simulink model "temp_mmms4th"  (R2024b)
settings: Solver=VariableStepAuto  StartTime=0.0  StopTime=10.0  RelTol=1e-3
values from neighbouring files (symbols this model uses):
  iota0 = eye(6,6)    [Initiate_KUKA_inv.m]    (also in Main_MMMS.m; test_KUKA_elements.m)
  K_d = 10*[1.3*eye(3) zeros(3);zeros(3) 0.8*eye(3)]    [Initiate_FQ.m]    (also in Initiate_KUKA_inv.m = 5*[0.7*eye(3) zeros(3);zeros(3) 0.5*eye(3)]; MMMS_Initiate_FQ.m; Main_MMMS.m = 5*[0.7*eye(3) zeros(3);zeros(3) 0.5*eye(3)]; test_KUKA_elements.m = 50*[0.7*eye(3) zeros(3);zeros(3) 0.5*eye(3)])
  K_i = 5*[0.1*eye(3) zeros(3);zeros(3) 0.01*eye(3)]    [Initiate_FQ.m]    (also in Initiate_KUKA_inv.m = 5*[0.01*eye(3) zeros(3);zeros(3) 0.001*eye(3)]; MMMS_Initiate_FQ.m; Main_MMMS.m = 5*[0.01*eye(3) zeros(3);zeros(3) 0.001*eye(3)]; test_KUKA_elements.m = 50*[0.01*eye(3) zeros(3);zeros(3) 0.001*eye(3)])
  K_p = 100*[0.1 0 0 0 0 0;0 0.1 0 0 0 0; 0 0 0.1 0 0 0; 0 0 0 0.01 0 0 ... (first row only)    [Initiate_FQ.m]    (also in Initiate_KUKA_inv.m = 5*[0.1 0 0 0 0 0;0 0.1 0 0 0 0; 0 0 0.1 0 0 0; 0 0 0 0.01 0 ; MMMS_Initiate_FQ.m; Main_MMMS.m = 5*[0.1 0 0 0 0 0;0 0.1 0 0 0 0; 0 0 0.1 0 0 0; 0 0 0 0.01 0 ; test_KUKA_elements.m = 50*[0.1 0 0 0 0 0;0 0.1 0 0 0 0; 0 0 0.1 0 0 0; 0 0 0 0.01 0)
  K_w = 200*eye(7)    [Initiate_FQ.m]    (also in MMMS_Initiate_FQ.m)
  K_wd = 2*eye(7)    [Initiate_FQ.m]    (also in MMMS_Initiate_FQ.m)
  M0 = M_temp.M0.data(:,:,1)    [Initiate_FQ.m]    (also in MMMS_Initiate_FQ.m; test_KUKA_elements.m)
  m0_frak = diag_M(1:6,1:6)    [Initiate_KUKA_inv.m]    (also in Main_MMMS.m; make_uncertain.m = diag_M_unc(1:6,1:6); test_KUKA_elements.m)
  M0m = M_temp.M0m.data(:,:,1)    [Initiate_FQ.m]    (also in MMMS_Initiate_FQ.m; test_KUKA_elements.m)
  m_diag = diag_M(7:end,7:end)    [Initiate_KUKA_inv.m]    (also in Main_MMMS.m; make_uncertain.m = diag_M_unc(7:end,7:end); test_KUKA_elements.m)
  M_t = (((Adjoint(g_It))'\M_t_body)/(Adjoint(g_It)))    [Initiate_FQ.m]    (also in Initiate_KUKA_inv.m = [eye(3)*mt zeros(3); zeros(3) eye(3)*80]; MMMS_Initiate_FQ.m; Main_MMMS.m = [eye(3)*mt zeros(3); zeros(3) eye(3)*80]; test_KUKA_elements.m = [eye(3)*mt zeros(3); zeros(3) eye(3)*80])
  M_t_body = [eye(3)*mt zeros(3); zeros(3) eye(3)*0.416667]    [Initiate_FQ.m]    (also in MMMS_Initiate_FQ.m)
  mu = P0    [Initiate_FQ.m]    (also in Initiate_KUKA_inv.m = zeros(6,1); MMMS_Initiate_FQ.m; Main_MMMS.m = zeros(6,1); make_uncertain.m = P0_unc)
  mu_t = inv((Adjoint(g_It))')*M_t_body*[V_It;w_t]    [Initiate_FQ.m]    (also in Initiate_KUKA_inv.m = M_t*[V_0t;w_t]; MMMS_Initiate_FQ.m; Main_MMMS.m = M_t*[V_0t;w_t]; make_uncertain.m = inv((Adjoint(g_It))')*M_t_body_unc*[V_It;w_t])
  sc_size = 1    [Initiate_KUKA_inv.m]    (also in Main_MMMS.m; test_KUKA_elements.m)
  Xi_m_matrix = zeros(6*n,n)    [Initiate_KUKA_inv.m]    (also in Main_MMMS.m)
undefined symbols (not defined in the file or in its folder): Mm, Xi_m
(part 1 of 2)
settings Model: Creator=bmonazza  LastModifiedBy=bmonazza

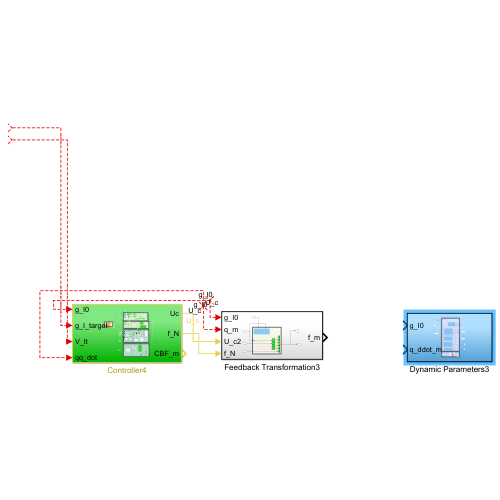
[thumbnail: Simulink's stored preview of the top-level diagram]
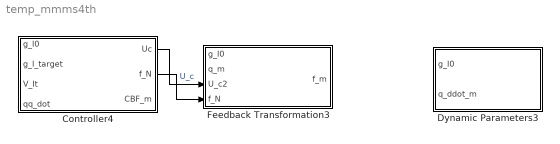
== system temp_mmms4th ==
  Controller4 : Subsystem
  Dynamic Parameters3 : Subsystem
  Feedback Transformation3 : Subsystem
  wires:
  ? -> Controller4/2(g_I_target)
  Controller4/1(Uc) -> Feedback Transformation3/3(U_c2)  "U_c"
  Controller4/2(f_N) -> Feedback Transformation3/4(f_N)
  ? -> Controller4/1(g_I0)  "g_I0"
  ? -> Feedback Transformation3/1(g_I0)  "g_I0"
  ? -> Feedback Transformation3/2(q_m)  "U_c"
  ? -> Controller4/3(V_It)
  ? -> Controller4/4(qq_dot)  "U_c"

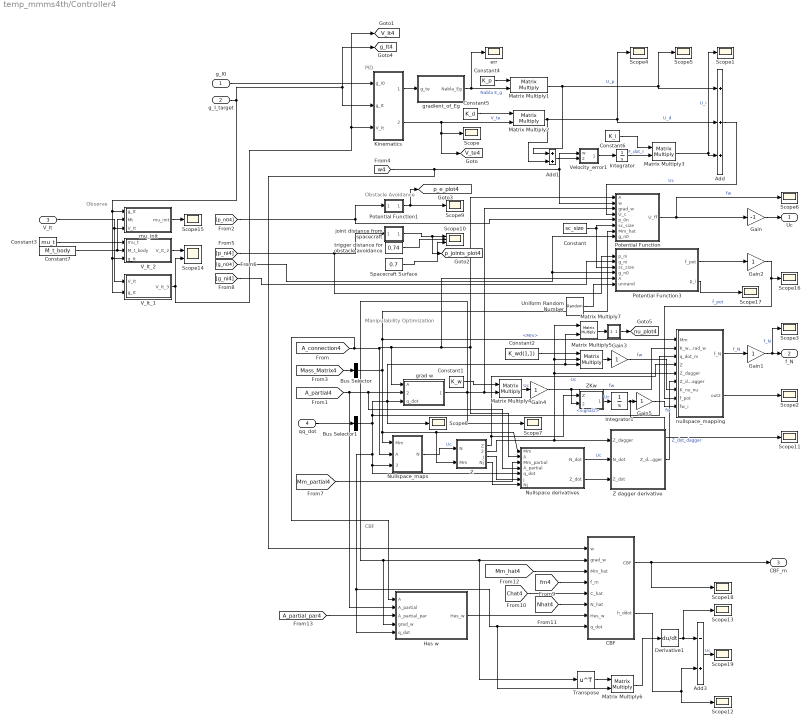
== system temp_mmms4th/Controller4 ==
  note: CBF
  note: Observe
  note: Obstacle Avoidance
  note: Manipulability Optimization
  note: PID
  g_I0 : Inport
  g_I_target : Inport  Port=2
  V_It : Inport  Port=3
  qq_dot : Inport  Port=4
  " " : MATLAB Function  TreatAsAtomicUnit=on
  Add : Sum  Inputs=+++
  Add1 : Sum
  Add3 : Sum  Inputs=-+
  Bus Selector : BusSelector  OutputSignals=Mm
  Bus Selector1 : BusSelector  OutputSignals=signal2
  CBF : MATLAB Function  TreatAsAtomicUnit=on
  Constant : Constant  Value=sc_size
  Constant1 : Constant  Value=K_w
  Constant2 : Constant  Value=K_wd(1,1)
  Constant3 : Constant  Value=mu_t
  Constant4 : Constant  Value=K_p
  Constant5 : Constant  Value=K_d
  Constant6 : Constant  Value=K_i
  Constant7 : Constant  Value=M_t_body
  Derivative1 : Derivative
  Gain : Gain  Gain=-1
  Gain{1..5} (5 alike) : Gain
  Hes w : MATLAB Function  TreatAsAtomicUnit=on
  Integrator : Integrator
  Integrator1 : Integrator
  Kinematics : Subsystem
  Matrix Multiply{1..4,6..7} (6 alike) : Product  Multiplication=Matrix(*)
  Matrix Multiply5 : Product  Inputs=3  Multiplication=Matrix(*)
  Nullspace derivatives : MATLAB Function  TreatAsAtomicUnit=on
  Nullspace_maps : MATLAB Function  TreatAsAtomicUnit=on
  Potential Function : MATLAB Function  TreatAsAtomicUnit=on
  Potential Function1 : MATLAB Function  TreatAsAtomicUnit=on
  Potential Function3 : MATLAB Function  TreatAsAtomicUnit=on
  Scope{,1..9,11..13,15..19} (18 alike) : Scope
  Scope10 : Scope  NumInputPorts=3
  Scope14 : Scope  NumInputPorts=2
  Spacecraft Surface : Constant  Value=0.7
  Transpose : Math  Operator=transpose
  Uniform Random Number : UniformRandomNumber  SampleTime=0.1
  V_It_1 : MATLAB Function  TreatAsAtomicUnit=on
  V_It_2 : MATLAB Function  TreatAsAtomicUnit=on
  Velocity_error1 : MATLAB Function  TreatAsAtomicUnit=on
  Z : MATLAB Function  TreatAsAtomicUnit=on
  Z dagger derivative : MATLAB Function  TreatAsAtomicUnit=on
  ZKw : MATLAB Function  TreatAsAtomicUnit=on
  err : Scope
  grad w : MATLAB Function  TreatAsAtomicUnit=on
  gradient_of_Eg : MATLAB Function  TreatAsAtomicUnit=on
  joint distance from spacecraft : MATLAB Function  TreatAsAtomicUnit=on
  mu_init : MATLAB Function  TreatAsAtomicUnit=on
  nullspace_mapping : MATLAB Function  TreatAsAtomicUnit=on
  trigger distance for obstacle avoidance : Constant  Value=0.74
  Uc : Outport
  f_N : Outport  Port=2
  CBF_m : Outport  Port=3
  tag scope: V_It4=global, V_te4=global, g_It4=global, nu_plot4=global, p_e_plot4=global, p_joints_plot4=global
  wires:
  Uniform Random Number/1 -> Potential Function3/6(unirand)
  [A_connection4] -> Hes w/1(A), Nullspace_maps/2(A), grad w/1(A), Nullspace derivatives/2(A), Potential Function/1(A), Potential Function3/5(A)
  [Chat4] -> CBF/5(C_hat)
  [Nhat4] -> CBF/6(N_hat)
  Derivative1/1 -> Add3/1, Scope13/1
  [A_partial_par4] -> Hes w/3(A_partial_par)
  Transpose/1 -> Matrix Multiply6/1
  Matrix Multiply6/1 -> Derivative1/1
  CBF/2(h_ddot) -> Scope12/1, Add3/2
  [Mm_hat4] -> CBF/3(Mm_hat)
  [fm4] -> CBF/4(f_m)
  Hes w/1(Hes_w) -> CBF/7(Hes_w)
  CBF/1(CBF) -> CBF_m/1, Scope18/1
  Add3/1 -> Scope19/1  "Uc"
  [w4] -> Velocity_error1/1(w), Potential Function/2(w), CBF/1(w)
  [A_partial4] -> Hes w/2(A_partial), Nullspace derivatives/4(A_partial), grad w/2(A_partial)
  Bus Selector1/1 -> Nullspace_maps/3(q_dot_m), Nullspace derivatives/5(q_dot), CBF/8(q_dot), Matrix Multiply6/2, Hes w/5(q_dot), Matrix Multiply5/3, Matrix Multiply7/2, grad w/3(q_dot), Scope8/1, nullspace_mapping/3(q_dot_m)  "<signal2>"
  grad w/1(grad_w) -> Matrix Multiply4/2, Potential Function/3(grad_w), Scope7/1, Hes w/4(grad_w), CBF/2(grad_w), Transpose/1
  Matrix Multiply7/1 -> " "/1(A)
  " "/1(normA) -> [nu_plot4]
  g_I_target/1 -> mu_init/1(g_It), V_It_2/3(g_It), V_It_1/2(g_It), [g_It4], Kinematics/2(g_It)
  Potential Function3/2(p_i) -> Scope17/1
  [g_ni4] -> Potential Function3/2(g_ni)
  Spacecraft Surface/1 -> Scope10/3
  V_It_1/1(V_It_3) -> [V_It4], Kinematics/3(V_It), Scope14/2
  V_It_2/1(V_It_2) -> Scope14/1
  Z/4(Nj) -> Nullspace derivatives/7(Nj)
  Z/3(j) -> Nullspace derivatives/6(j)
  Gain2/1 -> nullspace_mapping/8(f_pot), Scope16/1  "f_pot"
  Constant7/1 -> V_It_2/2(M_t_body), mu_init/2(Mt)
  mu_init/1(mu_init) -> Scope15/1
  Constant3/1 -> V_It_2/1(mu_t)
  V_It/1 -> mu_init/3(V_It), V_It_1/1(V_It)
  Gain5/1 -> nullspace_mapping/9(fw_i)  "fw"
  Integrator1/1 -> Gain5/1, Scope11/1
  ZKw/1(out) -> Integrator1/1  "Uc"
  Z/2(Z_dagger) -> Matrix Multiply5/2, Matrix Multiply7/1, nullspace_mapping/5(Z_dagger), Z dagger derivative/1(Z_dagger)
  nullspace_mapping/2(out2) -> Scope2/1
  Gain4/1 -> nullspace_mapping/2(K_w_grad_w), ZKw/2(K_w_grad_w)  "fw"
  Z/1(Z) -> nullspace_mapping/4(Z), ZKw/1(Z)  "Uc"
  [Mm_partial4] -> Nullspace derivatives/3(Mm_partial)
  Nullspace_maps/1(N) -> Z/1(N)  "Uc"
  Z dagger derivative/1(Z_dot_dagger) -> nullspace_mapping/6(Z_dot_dagger)  "Z_dot_dagger"
  Nullspace derivatives/2(Z_dot) -> Z dagger derivative/3(Z_dot)
  Nullspace derivatives/1(N_dot) -> Z dagger derivative/2(N_dot)  "Uc"
  Gain3/1 -> nullspace_mapping/7(K_nu_nu)  "fw"
  trigger distance for obstacle avoidance/1 -> Scope10/2
  Constant/1 -> Potential Function/6(sc_size), Potential Function3/3(sc_size)
  Potential Function3/1(f_pot) -> Gain2/1
  [g_n04] -> Potential Function/8(g_n0), Potential Function3/4(g_n0)
  joint distance from spacecraft/1(pnorm) -> Scope10/1, [p_joints_plot4]
  [p_ni4] -> Potential Function3/1(p_ni), joint distance from spacecraft/1(p_joints)
  Potential Function1/1(w_p) -> [p_e_plot4], Scope9/1
  [p_n04] -> Potential Function/5(p_0n), Potential Function1/1(p_0n)
  Velocity_error1/1(out) -> Integrator/1
  Potential Function/1(U_ff) -> Scope6/1, Gain/1  "fw"
  nullspace_mapping/1(f_N) -> Gain1/1  "f_N"
  Matrix Multiply3/1 -> Add/3, Scope1/1  "U_i"
  Matrix Multiply4/1 -> Gain4/1  "Uc"
  Constant2/1 -> Matrix Multiply5/1
  Matrix Multiply5/1 -> Gain3/1
  Constant1/1 -> Matrix Multiply4/1
  Gain1/1 -> Scope3/1, f_N/1  "f_N"
  Constant5/1 -> Matrix Multiply2/1
  Matrix Multiply1/1 -> Add1/1, Add/1, Scope5/1  "U_p"
  Integrator/1 -> Matrix Multiply3/2  "F_dot_I"
  Constant6/1 -> Matrix Multiply3/1
  Kinematics/2(V_te) -> Matrix Multiply2/2, Scope/1, [V_te4]  "V_te"
  Constant4/1 -> Matrix Multiply1/1
  gradient_of_Eg/1(Nabla_Eg) -> Matrix Multiply1/2, err/1  "Nabla E_g"
  Matrix Multiply2/1 -> Add1/2, Add/2, Scope4/1  "U_d"
  Add1/1 -> Velocity_error1/2(in)
  Kinematics/1(g_te1) -> gradient_of_Eg/1(g_te)
  Add/1 -> Potential Function/4(U_c)  "Uc"
  g_I0/1 -> Kinematics/1(g_I0)
  Gain/1 -> Uc/1
  Bus Selector/1 -> nullspace_mapping/1(Mm), Potential Function/7(Mm_hat), Nullspace derivatives/1(Mm), Z/2(Mm), Nullspace_maps/1(Mm)  "<Mm>"
  [Mass_Matrix4] -> Bus Selector/1
  qq_dot/1 -> Bus Selector1/1

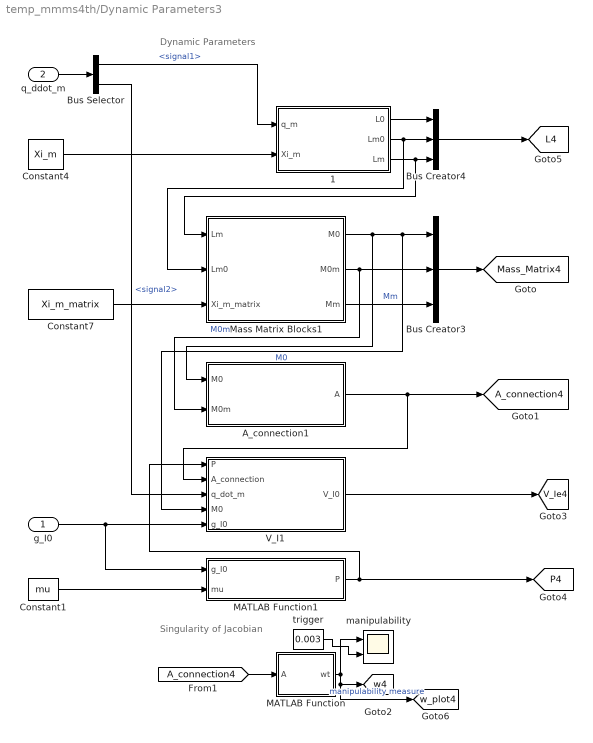
== system temp_mmms4th/Dynamic Parameters3 ==
  note: Dynamic Parameters
  note: Singularity of Jacobian
  g_I0 : Inport
  q_ddot_m : Inport  Port=2
  " 1" : MATLAB Function  TreatAsAtomicUnit=on
  A_connection1 : Subsystem
  Bus Creator3 : BusCreator  Inputs=M0,M0m,Mm
  Bus Creator4 : BusCreator  Inputs=3
  Bus Selector : BusSelector  OutputSignals=signal1,signal2
  Constant1 : Constant  Value=mu
  Constant4 : Constant  Value=Xi_m
  Constant7 : Constant  Value=Xi_m_matrix
  MATLAB Function : MATLAB Function  TreatAsAtomicUnit=on
  MATLAB Function1 : MATLAB Function  TreatAsAtomicUnit=on
  Mass Matrix Blocks1 : Subsystem
  V_I1 : MATLAB Function  TreatAsAtomicUnit=on
  manipulability : Scope  NumInputPorts=2
  trigger : Constant  Value=0.003
  tag scope: A_connection4=global, L4=global, Mass_Matrix4=global, P4=global, V_Ie4=global, w4=global, w_plot4=global
  wires:
  V_I1/1(V_I0) -> [V_Ie4]
  trigger/1 -> manipulability/2
  [A_connection4] -> MATLAB Function/1(A)
  MATLAB Function/1(wt) -> manipulability/1, [w4], [w_plot4]  "manipulability measure"
  Bus Selector/1 -> " 1"/1(q_m)  "<signal1>"
  Bus Selector/2 -> V_I1/3(q_dot_m)  "<signal2>"
  Mass Matrix Blocks1/2(M0m) -> A_connection1/2(M0m), Bus Creator3/2  "M0m"
  Constant7/1 -> Mass Matrix Blocks1/3(Xi_m_matrix)
  " 1"/3(Lm) -> Mass Matrix Blocks1/1(Lm), Bus Creator4/3
  Constant4/1 -> " 1"/2(Xi_m)
  " 1"/1(L0) -> Bus Creator4/1
  " 1"/2(Lm0) -> Bus Creator4/2, Mass Matrix Blocks1/2(Lm0)
  q_ddot_m/1 -> Bus Selector/1
  Bus Creator4/1 -> [L4]
  Bus Creator3/1 -> [Mass_Matrix4]
  Mass Matrix Blocks1/3(Mm) -> Bus Creator3/3  "Mm"
  Mass Matrix Blocks1/1(M0) -> Bus Creator3/1, V_I1/4(M0), A_connection1/1(M0)  "M0"
  A_connection1/1(A) -> V_I1/2(A_connection), [A_connection4]
  g_I0/1 -> V_I1/5(g_I0), MATLAB Function1/1(g_I0)
  Constant1/1 -> MATLAB Function1/2(mu)
  MATLAB Function1/1(P) -> [P4], V_I1/1(P)

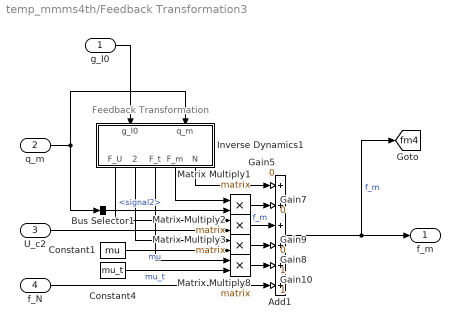
== system temp_mmms4th/Feedback Transformation3 ==
  note: Feedback Transformation
  g_I0 : Inport
  q_m : Inport  Port=2
  U_c2 : Inport  Port=3
  f_N : Inport  Port=4
  Add1 : Sum  Inputs=++++++
  Bus Selector1 : BusSelector  OutputSignals=signal2
  Constant1 : Constant  Value=mu
  Constant4 : Constant  Value=mu_t
  Gain10 : Gain
  Gain5 : Gain  Gain=0
  Gain7 : Gain  Gain=0
  Gain8 : Gain
  Gain9 : Gain  Gain=0
  Inverse Dynamics1 : Subsystem
  Matrix Multiply{1..3,8} (4 alike) : Product  Multiplication=Matrix(*)
  f_m : Outport
  tag scope: fm4=global
  wires:
  q_m/1 -> Inverse Dynamics1/2("q_m "), Bus Selector1/1
  g_I0/1 -> Inverse Dynamics1/1(g_I0)
  Gain8/1 -> Add1/5
  Inverse Dynamics1/3(F_t) -> Matrix Multiply8/1
  Inverse Dynamics1/4(F_m) -> Matrix Multiply1/1
  Gain9/1 -> Add1/4
  Constant4/1 -> Matrix Multiply8/2  "mu_t"
  Add1/1 -> f_m/1, [fm4]  "f_m"
  Bus Selector1/1 -> Matrix Multiply1/2  "<signal2>"
  Matrix Multiply2/1 -> Add1/3  "f_m"
  f_N/1 -> Gain10/1
  Gain5/1 -> Add1/1
  Matrix Multiply3/1 -> Gain9/1
  Matrix Multiply8/1 -> Gain8/1
  Inverse Dynamics1/5(N) -> Gain5/1
  U_c2/1 -> Matrix Multiply2/2
  Constant1/1 -> Matrix Multiply3/2  "mu"
  Inverse Dynamics1/1(F_U) -> Matrix Multiply2/1
  Gain10/1 -> Add1/6
  Matrix Multiply1/1 -> Gain7/1
  Gain7/1 -> Add1/2
  Inverse Dynamics1/2(F_mu) -> Matrix Multiply3/1

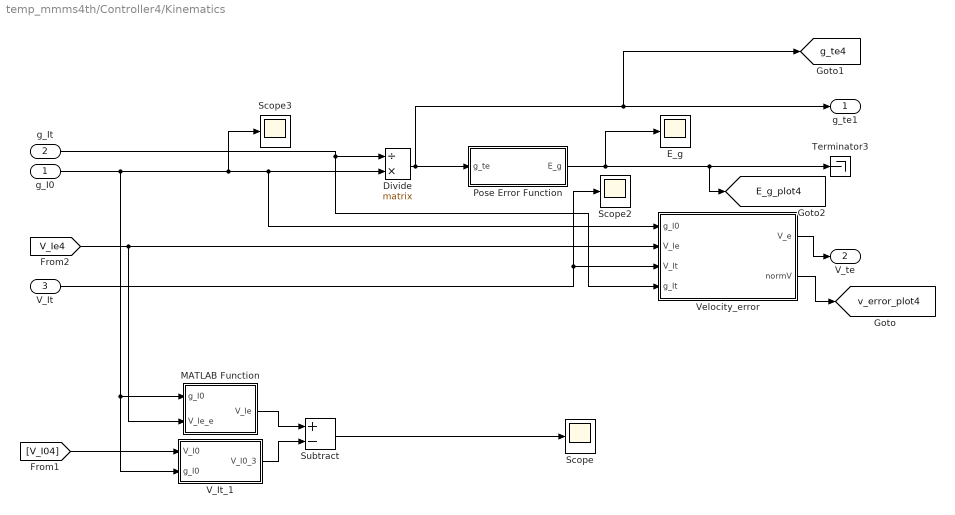
== system temp_mmms4th/Controller4/Kinematics ==
  g_I0 : Inport
  g_It : Inport  Port=2
  V_It : Inport  Port=3
  Divide : Product  Inputs=/*  Multiplication=Matrix(*)
  E_g : Scope
  MATLAB Function : MATLAB Function  TreatAsAtomicUnit=on
  Pose Error Function : MATLAB Function  TreatAsAtomicUnit=on
  Scope : Scope
  Scope2 : Scope
  Scope3 : Scope
  Subtract : Sum  Inputs=+-
  Terminator3 : Terminator
  V_It_1 : MATLAB Function  TreatAsAtomicUnit=on
  Velocity_error : MATLAB Function  TreatAsAtomicUnit=on
  g_te1 : Outport
  V_te : Outport  Port=2
  tag scope: E_g_plot4=global, g_te4=global, v_error_plot4=global
  wires:
  Velocity_error/2(normV) -> [v_error_plot4]
  V_It_1/1(V_I0_3) -> Subtract/2
  MATLAB Function/1(V_Ie) -> Subtract/1
  Subtract/1 -> Scope/1
  [V_I04] -> V_It_1/1(V_I0)
  Pose Error Function/1(E_g) -> Terminator3/1, [E_g_plot4], E_g/1
  [V_Ie4] -> Velocity_error/2(V_Ie), MATLAB Function/2(V_Ie_e)
  V_It/1 -> Scope2/1, Velocity_error/3(V_It)
  Velocity_error/1(V_e) -> V_te/1
  Divide/1 -> Pose Error Function/1(g_te), [g_te4], g_te1/1
  g_I0/1 -> Divide/2, Velocity_error/1(g_I0), Scope3/1, V_It_1/2(g_I0), MATLAB Function/1(g_I0)
  g_It/1 -> Divide/1, Velocity_error/4(g_It)

== system temp_mmms4th/Dynamic Parameters3/A_connection1 ==
  M0 : Inport
  M0m : Inport  Port=2
  Divide : Product  Inputs=/*  Multiplication=Matrix(*)
  A : Outport
  wires:
  M0m/1 -> Divide/2
  M0/1 -> Divide/1
  Divide/1 -> A/1

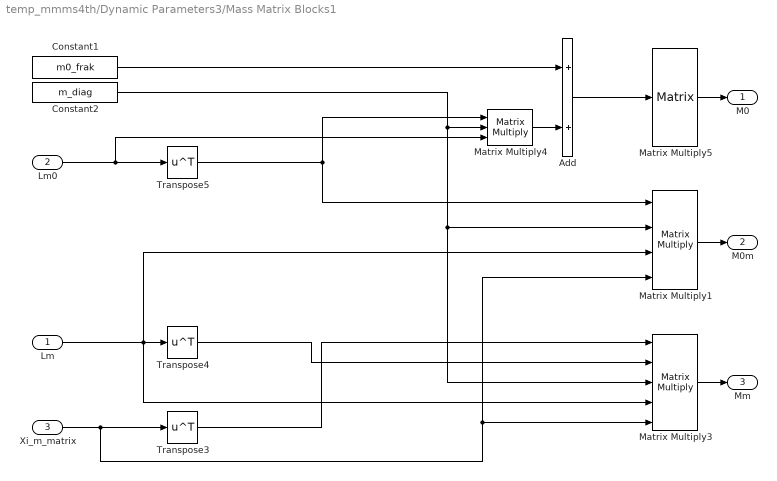
== system temp_mmms4th/Dynamic Parameters3/Mass Matrix Blocks1 ==
  Lm : Inport
  Lm0 : Inport  Port=2
  Xi_m_matrix : Inport  Port=3
  Add : Sum
  Constant1 : Constant  Value=m0_frak  VectorParams1D=off
  Constant2 : Constant  Value=m_diag  VectorParams1D=off
  Matrix Multiply1 : Product  Inputs=4  Multiplication=Matrix(*)
  Matrix Multiply3 : Product  Inputs=5  Multiplication=Matrix(*)
  Matrix Multiply4 : Product  Inputs=3  Multiplication=Matrix(*)
  Matrix Multiply5 : Product  Inputs=1  Multiplication=Matrix(*)
  Transpose3 : Math  Operator=transpose
  Transpose4 : Math  Operator=transpose
  Transpose5 : Math  Operator=transpose
  M0 : Outport
  M0m : Outport  Port=2
  Mm : Outport  Port=3
  wires:
  Constant1/1 -> Add/1
  Constant2/1 -> Matrix Multiply1/2, Matrix Multiply3/3, Matrix Multiply4/2
  Add/1 -> Matrix Multiply5/1
  Lm/1 -> Transpose4/1, Matrix Multiply3/4, Matrix Multiply1/3
  Transpose3/1 -> Matrix Multiply3/1
  Matrix Multiply4/1 -> Add/2
  Matrix Multiply1/1 -> M0m/1
  Matrix Multiply3/1 -> Mm/1
  Transpose4/1 -> Matrix Multiply3/2
  Transpose5/1 -> Matrix Multiply1/1, Matrix Multiply4/1
  Lm0/1 -> Matrix Multiply4/3, Transpose5/1
  Matrix Multiply5/1 -> M0/1
  Xi_m_matrix/1 -> Transpose3/1, Matrix Multiply3/5, Matrix Multiply1/4

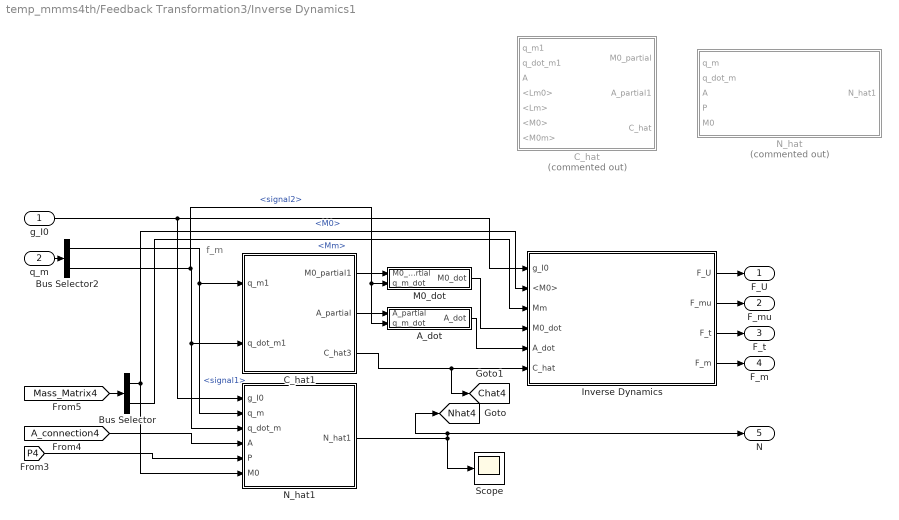
== system temp_mmms4th/Feedback Transformation3/Inverse Dynamics1 ==
  note: f_m
  g_I0 : Inport
  "q_m " : Inport  Port=2
  A_dot : MATLAB Function  TreatAsAtomicUnit=on
  Bus Selector : BusSelector  OutputSignals=M0,Mm
  Bus Selector2 : BusSelector  OutputSignals=signal1,signal2
  C_hat : Subsystem  Commented=on
  C_hat1 : Subsystem
  Inverse Dynamics : Subsystem
  M0_dot : MATLAB Function  TreatAsAtomicUnit=on
  N_hat : Subsystem  Commented=on
  N_hat1 : Subsystem
  Scope : Scope
  F_U : Outport
  F_mu : Outport  Port=2
  F_t : Outport  Port=3
  F_m : Outport  Port=4
  N : Outport  Port=5
  tag scope: Chat4=global, Nhat4=global
  wires:
  C_hat1/3(C_hat3) -> Inverse Dynamics/6(C_hat), [Chat4]
  N_hat1/1(N_hat1) -> Scope/1, [Nhat4], N/1
  [A_connection4] -> N_hat1/4(A)
  "q_m "/1 -> Bus Selector2/1
  A_dot/1(A_dot) -> Inverse Dynamics/5(A_dot)
  M0_dot/1(M0_dot) -> Inverse Dynamics/4(M0_dot)
  C_hat1/2(A_partial) -> A_dot/1(A_partial)
  C_hat1/1(M0_partial1) -> M0_dot/1(M0_partial)
  Bus Selector2/2 -> N_hat1/3(q_dot_m), C_hat1/2(q_dot_m1), M0_dot/2(q_m_dot), A_dot/2(q_m_dot)  "<signal2>"
  Bus Selector2/1 -> N_hat1/2(q_m), C_hat1/1(q_m1)  "<signal1>"
  Bus Selector/2 -> Inverse Dynamics/3(Mm)  "<Mm>"
  Inverse Dynamics/4(F_m) -> F_m/1
  Inverse Dynamics/3(F_t) -> F_t/1
  Inverse Dynamics/2(F_mu) -> F_mu/1
  Inverse Dynamics/1(F_U) -> F_U/1
  g_I0/1 -> Inverse Dynamics/1(g_I0), N_hat1/1(g_I0)
  Bus Selector/1 -> Inverse Dynamics/2(<M0>), N_hat1/6(M0)  "<M0>"
  [Mass_Matrix4] -> Bus Selector/1
  [P4] -> N_hat1/5(P)

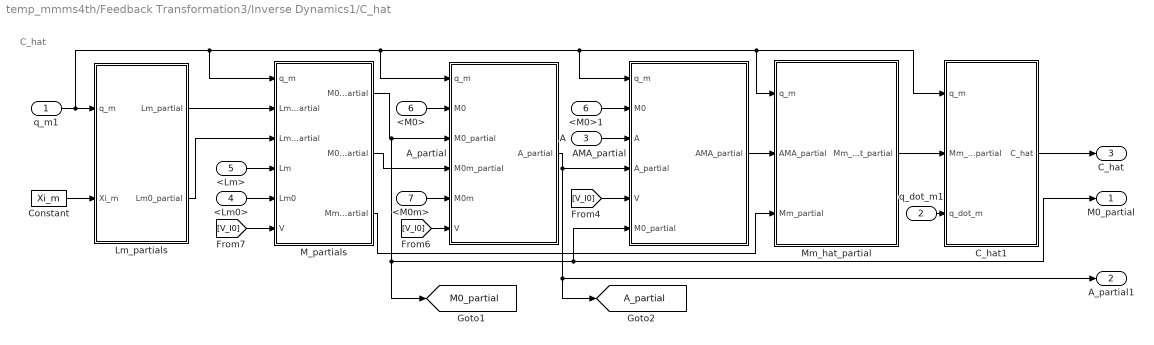
== system temp_mmms4th/Feedback Transformation3/Inverse Dynamics1/C_hat ==
  note: C_hat
  q_m1 : Inport
  q_dot_m1 : Inport  Port=2
  A : Inport  Port=3
  <Lm0> : Inport  Port=4
  <Lm> : Inport  Port=5
  <M0> : Inport  Port=6
  <M0m> : Inport  Port=7
  <M0>1 : InportShadow  Port=6
  AMA_partial : MATLAB Function  TreatAsAtomicUnit=on
  A_partial : MATLAB Function  TreatAsAtomicUnit=on
  C_hat1 : MATLAB Function  TreatAsAtomicUnit=on
  Constant : Constant  Value=Xi_m
  Lm_partials : Subsystem
  M_partials : Subsystem
  Mm_hat_partial : MATLAB Function  TreatAsAtomicUnit=on
  M0_partial : Outport
  A_partial1 : Outport  Port=2
  C_hat : Outport  Port=3
  tag scope: A_partial=global, M0_partial=global
  wires:
  <Lm0>/1 -> M_partials/5(Lm0)
  <M0>1/1 -> AMA_partial/2(M0)
  C_hat1/1(C_hat) -> C_hat/1
  A/1 -> AMA_partial/3(A)
  [V_I0] -> AMA_partial/5(V)
  <Lm>/1 -> M_partials/4(Lm)
  [V_I0] -> M_partials/6(V)
  [V_I0] -> A_partial/6(V)
  <M0>/1 -> A_partial/2(M0)
  AMA_partial/1(AMA_partial) -> Mm_hat_partial/2(AMA_partial)
  q_dot_m1/1 -> C_hat1/3(q_dot_m)
  Mm_hat_partial/1(Mm_hat_partial) -> C_hat1/2(Mm_hat_partial)
  M_partials/2(M0m_partial) -> A_partial/4(M0m_partial)
  Constant/1 -> Lm_partials/2(Xi_m)
  A_partial/1(A_partial) -> A_partial1/1, [A_partial], AMA_partial/4(A_partial)
  M_partials/1(M0_partial) -> [M0_partial], AMA_partial/6(M0_partial), M0_partial/1, A_partial/3(M0_partial)
  Lm_partials/1(Lm_partial) -> M_partials/2(Lm_partial)
  <M0m>/1 -> A_partial/5(M0m)
  q_m1/1 -> M_partials/1(q_m), A_partial/1(q_m), AMA_partial/1(q_m), C_hat1/1(q_m), Mm_hat_partial/1(q_m), Lm_partials/1(q_m)
  Lm_partials/2(Lm0_partial) -> M_partials/3(Lm0_partial)
  M_partials/3(Mm_partial) -> Mm_hat_partial/3(Mm_partial)

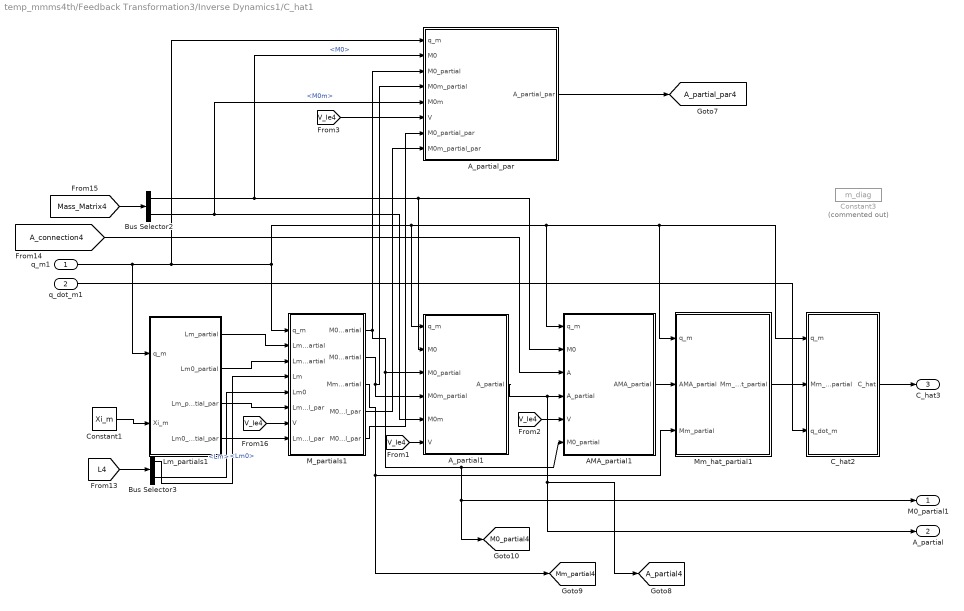
== system temp_mmms4th/Feedback Transformation3/Inverse Dynamics1/C_hat1 ==
  q_m1 : Inport
  q_dot_m1 : Inport  Port=2
  AMA_partial1 : MATLAB Function  TreatAsAtomicUnit=on
  A_partial1 : MATLAB Function  TreatAsAtomicUnit=on
  A_partial_par : MATLAB Function  TreatAsAtomicUnit=on
  Bus Selector2 : BusSelector  OutputSignals=M0,M0m
  Bus Selector3 : BusSelector  OutputSignals=Lm,Lm0
  C_hat2 : MATLAB Function  TreatAsAtomicUnit=on
  Constant1 : Constant  Value=Xi_m
  Constant3 : Constant  Commented=on  Value=m_diag  VectorParams1D=off
  Lm_partials1 : Subsystem
  M_partials1 : Subsystem
  Mm_hat_partial1 : MATLAB Function  TreatAsAtomicUnit=on
  M0_partial1 : Outport
  A_partial : Outport  Port=2
  C_hat3 : Outport  Port=3
  tag scope: A_partial4=global, A_partial_par4=global, M0_partial4=global, Mm_partial4=global
  wires:
  Lm_partials1/4(Lm0_partial_par) -> M_partials1/8(Lm0_partial_par)
  M_partials1/4(M0m_partial_par) -> A_partial_par/8(M0m_partial_par)
  Bus Selector3/2 -> M_partials1/5(Lm0)  "<Lm0>"
  Bus Selector3/1 -> M_partials1/4(Lm)  "<Lm>"
  M_partials1/5(M0_partial_par) -> A_partial_par/7(M0_partial_par)
  M_partials1/3(Mm_partial) -> Mm_hat_partial1/3(Mm_partial), [Mm_partial4]
  AMA_partial1/1(AMA_partial) -> Mm_hat_partial1/2(AMA_partial)
  q_dot_m1/1 -> C_hat2/3(q_dot_m)
  [V_Ie4] -> A_partial1/6(V)
  [L4] -> Bus Selector3/1
  A_partial1/1(A_partial) -> AMA_partial1/4(A_partial), A_partial/1, [A_partial4]
  q_m1/1 -> Lm_partials1/1(q_m), M_partials1/1(q_m), A_partial1/1(q_m), Mm_hat_partial1/1(q_m), C_hat2/1(q_m), AMA_partial1/1(q_m), A_partial_par/1(q_m)
  Lm_partials1/3(Lm_partial_par) -> M_partials1/6(Lm_partial_par)
  M_partials1/1(M0_partial) -> A_partial_par/3(M0_partial), A_partial1/3(M0_partial), M0_partial1/1, [M0_partial4], AMA_partial1/6(M0_partial)
  Lm_partials1/2(Lm0_partial) -> M_partials1/3(Lm0_partial)
  Constant1/1 -> Lm_partials1/2(Xi_m)
  [V_Ie4] -> M_partials1/7(V)
  Bus Selector2/2 -> A_partial1/5(M0m), A_partial_par/5(M0m)  "<M0m>"
  [A_connection4] -> AMA_partial1/3(A)
  [Mass_Matrix4] -> Bus Selector2/1
  Bus Selector2/1 -> A_partial1/2(M0), AMA_partial1/2(M0), A_partial_par/2(M0)  "<M0>"
  M_partials1/2(M0m_partial) -> A_partial1/4(M0m_partial), A_partial_par/4(M0m_partial)
  Mm_hat_partial1/1(Mm_hat_partial) -> C_hat2/2(Mm_hat_partial)
  [V_Ie4] -> A_partial_par/6(V)
  Lm_partials1/1(Lm_partial) -> M_partials1/2(Lm_partial)
  [V_Ie4] -> AMA_partial1/5(V)
  A_partial_par/1(A_partial_par) -> [A_partial_par4]
  C_hat2/1(C_hat) -> C_hat3/1

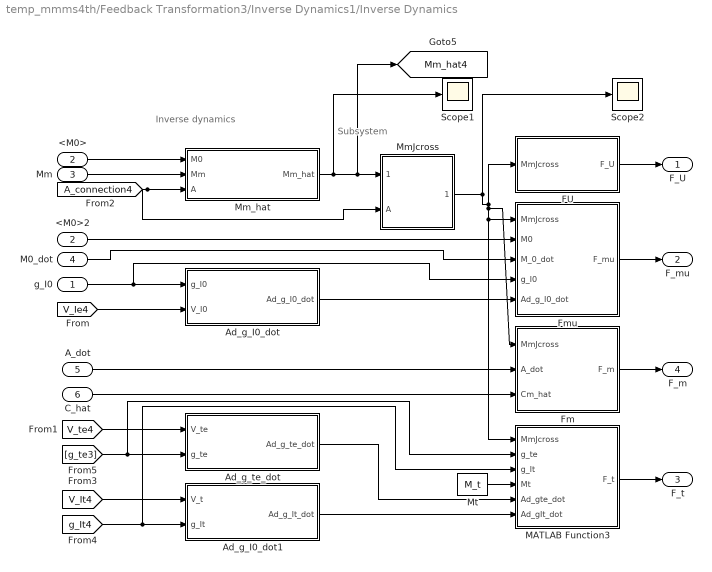
== system temp_mmms4th/Feedback Transformation3/Inverse Dynamics1/Inverse Dynamics ==
  note: Inverse dynamics
  note: Subsystem
  g_I0 : Inport
  <M0> : Inport  Port=2
  Mm : Inport  Port=3
  M0_dot : Inport  Port=4
  A_dot : Inport  Port=5
  C_hat : Inport  Port=6
  <M0>2 : InportShadow  Port=2
  Ad_g_I0_dot : MATLAB Function  TreatAsAtomicUnit=on
  Ad_g_I0_dot1 : MATLAB Function  TreatAsAtomicUnit=on
  Ad_g_te_dot : MATLAB Function  TreatAsAtomicUnit=on
  FU : MATLAB Function  TreatAsAtomicUnit=on
  Fm : MATLAB Function  TreatAsAtomicUnit=on
  Fmu : MATLAB Function  TreatAsAtomicUnit=on
  MATLAB Function3 : MATLAB Function  TreatAsAtomicUnit=on
  MmJcross : MATLAB Function  TreatAsAtomicUnit=on
  Mm_hat : MATLAB Function  TreatAsAtomicUnit=on
  Mt : Constant  Value=M_t
  Scope1 : Scope
  Scope2 : Scope
  F_U : Outport
  F_mu : Outport  Port=2
  F_t : Outport  Port=3
  F_m : Outport  Port=4
  tag scope: Mm_hat4=global
  wires:
  Mm_hat/1(Mm_hat) -> Scope1/1, MmJcross/1(Mm_hat), [Mm_hat4]
  MmJcross/1(MmJcross) -> Scope2/1, Fm/1(MmJcross), Fmu/1(MmJcross), MATLAB Function3/1(MmJcross), FU/1(MmJcross)
  Mt/1 -> MATLAB Function3/4(Mt)
  [V_It4] -> Ad_g_I0_dot1/1(V_t)
  [V_te4] -> Ad_g_te_dot/1(V_te)
  [g_It4] -> Ad_g_I0_dot1/2(g_It), MATLAB Function3/3(g_It)
  [g_te3] -> Ad_g_te_dot/2(g_te), MATLAB Function3/2(g_te)
  Ad_g_te_dot/1(Ad_g_te_dot) -> MATLAB Function3/5(Ad_gte_dot)
  Ad_g_I0_dot/1(Ad_g_I0_dot) -> Fmu/5(Ad_g_I0_dot)
  Ad_g_I0_dot1/1(Ad_g_It_dot) -> MATLAB Function3/6(Ad_gIt_dot)
  [V_Ie4] -> Ad_g_I0_dot/2(V_I0)
  A_dot/1 -> Fm/2(A_dot)
  M0_dot/1 -> Fmu/3(M_0_dot)
  g_I0/1 -> Ad_g_I0_dot/1(g_I0), Fmu/4(g_I0)
  <M0>2/1 -> Fmu/2(M0)
  C_hat/1 -> Fm/3(Cm_hat)
  <M0>/1 -> Mm_hat/1(M0)
  Fm/1(F_m) -> F_m/1
  MATLAB Function3/1(F_t) -> F_t/1
  Fmu/1(F_mu) -> F_mu/1
  FU/1(F_U) -> F_U/1
  [A_connection4] -> MmJcross/2(A), Mm_hat/3(A)
  Mm/1 -> Mm_hat/2(Mm)

== system temp_mmms4th/Feedback Transformation3/Inverse Dynamics1/N_hat ==
  q_m : Inport
  q_dot_m : Inport  Port=2
  A : Inport  Port=3
  P : Inport  Port=4
  M0 : Inport  Port=5
  Constant : Constant  Value=iota0
  Matrix Multiply : Product  Multiplication=Matrix(*)
  N_hat : MATLAB Function  TreatAsAtomicUnit=on
  To Workspace : ToWorkspace  VariableName=N_firstpart  SaveFormat=Timeseries  SampleTime=-1
  N_hat1 : Outport
  wires:
  M0/1 -> N_hat/9(M0)
  Matrix Multiply/1 -> N_hat1/1
  Constant/1 -> N_hat/8(iota0)
  [A_partial] -> N_hat/7(A_partial)
  A/1 -> N_hat/3(A)
  [V_I0] -> N_hat/4(V)
  q_dot_m/1 -> N_hat/2(q_dot_m)
  q_m/1 -> N_hat/1(q_m)
  N_hat/1(N_hat_temp) -> Matrix Multiply/1, To Workspace/1
  [M0_partial] -> N_hat/6(M0_partial)
  P/1 -> N_hat/5(P), Matrix Multiply/2

== system temp_mmms4th/Feedback Transformation3/Inverse Dynamics1/N_hat1 ==
  g_I0 : Inport
  q_m : Inport  Port=2
  q_dot_m : Inport  Port=3
  A : Inport  Port=4
  P : Inport  Port=5
  M0 : Inport  Port=6
  Constant : Constant  Value=iota0
  MATLAB Function : MATLAB Function  TreatAsAtomicUnit=on
  Matrix Multiply : Product  Multiplication=Matrix(*)
  N_hat : MATLAB Function  TreatAsAtomicUnit=on
  N_hat1 : Outport
  wires:
  g_I0/1 -> MATLAB Function/1(g_I0)
  MATLAB Function/1(V_Ie) -> N_hat/4(V)
  P/1 -> N_hat/5(P), Matrix Multiply/2
  M0/1 -> N_hat/9(M0)
  Matrix Multiply/1 -> N_hat1/1
  Constant/1 -> N_hat/8(iota0)
  [A_partial4] -> N_hat/7(A_partial)
  A/1 -> N_hat/3(A)
  [V_Ie4] -> MATLAB Function/2(V_Ie_e)
  q_dot_m/1 -> N_hat/2(q_dot_m)
  q_m/1 -> N_hat/1(q_m)
  N_hat/1(N_hat_temp) -> Matrix Multiply/1
  [M0_partial4] -> N_hat/6(M0_partial)

== system temp_mmms4th/Feedback Transformation3/Inverse Dynamics1/C_hat/Lm_partials ==
  q_m : Inport
  Xi_m : Inport  Port=2
  Constant : Constant  Value=iota0
  Lm0partial : MATLAB Function  TreatAsAtomicUnit=on
  Lmpartial : MATLAB Function  TreatAsAtomicUnit=on
  Lm_partial : Outport
  Lm0_partial : Outport  Port=2
  wires:
  Xi_m/1 -> Lmpartial/2(Xi_m), Lm0partial/2(Xi_m)
  q_m/1 -> Lmpartial/1(q_m), Lm0partial/1(q_m)
  Constant/1 -> Lmpartial/3(iota0), Lm0partial/3(iota0)
  Lm0partial/1(Lm0_partial) -> Lm0_partial/1
  Lmpartial/1(Lm_partial) -> Lm_partial/1

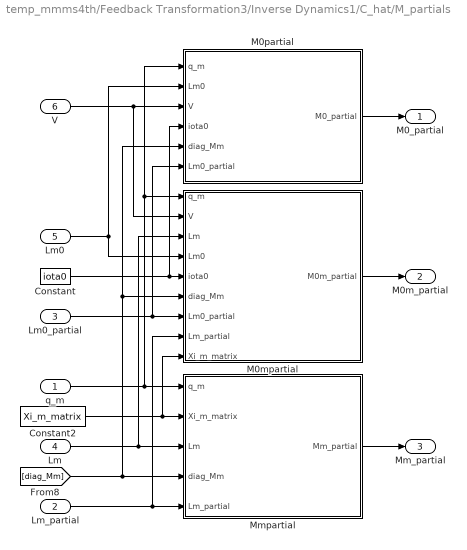
== system temp_mmms4th/Feedback Transformation3/Inverse Dynamics1/C_hat/M_partials ==
  q_m : Inport
  Lm_partial : Inport  Port=2
  Lm0_partial : Inport  Port=3
  Lm : Inport  Port=4
  Lm0 : Inport  Port=5
  V : Inport  Port=6
  " M0partial" : MATLAB Function  TreatAsAtomicUnit=on
  Constant : Constant  Value=iota0
  Constant2 : Constant  Value=Xi_m_matrix
  M0mpartial : MATLAB Function  TreatAsAtomicUnit=on
  Mmpartial : MATLAB Function  TreatAsAtomicUnit=on
  M0_partial : Outport
  M0m_partial : Outport  Port=2
  Mm_partial : Outport  Port=3
  wires:
  V/1 -> " M0partial"/3(V), M0mpartial/2(V)
  Constant/1 -> M0mpartial/5(iota0), " M0partial"/4(iota0)
  Lm0_partial/1 -> M0mpartial/7(Lm0_partial), " M0partial"/6(Lm0_partial)
  Lm0/1 -> " M0partial"/2(Lm0), M0mpartial/4(Lm0)
  " M0partial"/1(M0_partial) -> M0_partial/1
  M0mpartial/1(M0m_partial) -> M0m_partial/1
  Mmpartial/1(Mm_partial) -> Mm_partial/1
  Lm/1 -> Mmpartial/3(Lm), M0mpartial/3(Lm)
  Constant2/1 -> Mmpartial/2(Xi_m_matrix), M0mpartial/9(Xi_m_matrix)
  [diag_Mm] -> Mmpartial/4(diag_Mm), M0mpartial/6(diag_Mm), " M0partial"/5(diag_Mm)
  q_m/1 -> Mmpartial/1(q_m), M0mpartial/1(q_m), " M0partial"/1(q_m)
  Lm_partial/1 -> Mmpartial/5(Lm_partial), M0mpartial/8(Lm_partial)

== system temp_mmms4th/Feedback Transformation3/Inverse Dynamics1/C_hat1/Lm_partials1 ==
  q_m : Inport
  Xi_m : Inport  Port=2
  Constant : Constant  Value=iota0
  Lm0partial : MATLAB Function  TreatAsAtomicUnit=on
  Lm0partial_par : MATLAB Function  TreatAsAtomicUnit=on
  Lmpartial : MATLAB Function  TreatAsAtomicUnit=on
  Lmpartial_par : MATLAB Function  TreatAsAtomicUnit=on
  Lm_partial : Outport
  Lm0_partial : Outport  Port=2
  Lm_partial_par : Outport  Port=3
  Lm0_partial_par : Outport  Port=4
  wires:
  Lmpartial_par/1(Lm_partial_par) -> Lm_partial_par/1
  Lm0partial_par/1(Lm0_partial_par) -> Lm0_partial_par/1
  Xi_m/1 -> Lmpartial/2(Xi_m), Lm0partial/2(Xi_m), Lmpartial_par/2(Xi_m), Lm0partial_par/2(Xi_m)
  q_m/1 -> Lmpartial/1(q_m), Lm0partial/1(q_m), Lmpartial_par/1(q_m), Lm0partial_par/1(q_m)
  Constant/1 -> Lmpartial/3(iota0), Lm0partial/3(iota0), Lmpartial_par/3(iota0), Lm0partial_par/3(iota0)
  Lm0partial/1(Lm0_partial) -> Lm0_partial/1
  Lmpartial/1(Lm_partial) -> Lm_partial/1

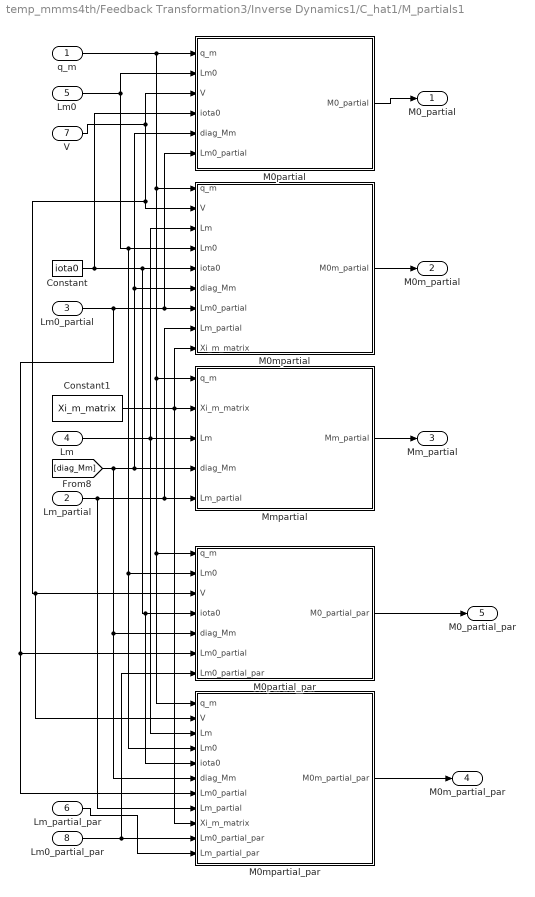
== system temp_mmms4th/Feedback Transformation3/Inverse Dynamics1/C_hat1/M_partials1 ==
  q_m : Inport
  Lm_partial : Inport  Port=2
  Lm0_partial : Inport  Port=3
  Lm : Inport  Port=4
  Lm0 : Inport  Port=5
  Lm_partial_par : Inport  Port=6
  V : Inport  Port=7
  Lm0_partial_par : Inport  Port=8
  " M0partial" : MATLAB Function  TreatAsAtomicUnit=on
  " M0partial_par" : MATLAB Function  TreatAsAtomicUnit=on
  Constant : Constant  Value=iota0
  Constant1 : Constant  Value=Xi_m_matrix
  M0mpartial : MATLAB Function  TreatAsAtomicUnit=on
  M0mpartial_par : MATLAB Function  TreatAsAtomicUnit=on
  Mmpartial : MATLAB Function  TreatAsAtomicUnit=on
  M0_partial : Outport
  M0m_partial : Outport  Port=2
  Mm_partial : Outport  Port=3
  M0m_partial_par : Outport  Port=4
  M0_partial_par : Outport  Port=5
  wires:
  Lm_partial_par/1 -> M0mpartial_par/11(Lm_partial_par)
  Lm0_partial_par/1 -> M0mpartial_par/10(Lm0_partial_par), " M0partial_par"/7(Lm0_partial_par)
  " M0partial_par"/1(M0_partial_par) -> M0_partial_par/1
  M0mpartial_par/1(M0m_partial_par) -> M0m_partial_par/1
  V/1 -> " M0partial"/3(V), M0mpartial/2(V), " M0partial_par"/3(V), M0mpartial_par/2(V)
  Constant/1 -> " M0partial"/4(iota0), M0mpartial/5(iota0), " M0partial_par"/4(iota0), M0mpartial_par/5(iota0)
  Lm0_partial/1 -> M0mpartial/7(Lm0_partial), " M0partial"/6(Lm0_partial), M0mpartial_par/7(Lm0_partial), " M0partial_par"/6(Lm0_partial)
  Lm0/1 -> M0mpartial/4(Lm0), " M0partial_par"/2(Lm0), M0mpartial_par/4(Lm0), " M0partial"/2(Lm0)
  " M0partial"/1(M0_partial) -> M0_partial/1
  M0mpartial/1(M0m_partial) -> M0m_partial/1
  Mmpartial/1(Mm_partial) -> Mm_partial/1
  Lm/1 -> Mmpartial/3(Lm), M0mpartial/3(Lm), M0mpartial_par/3(Lm)
  Constant1/1 -> Mmpartial/2(Xi_m_matrix), M0mpartial/9(Xi_m_matrix), M0mpartial_par/9(Xi_m_matrix)
  [diag_Mm] -> Mmpartial/4(diag_Mm), M0mpartial/6(diag_Mm), " M0partial"/5(diag_Mm), " M0partial_par"/5(diag_Mm), M0mpartial_par/6(diag_Mm)
  q_m/1 -> " M0partial"/1(q_m), M0mpartial/1(q_m), Mmpartial/1(q_m), " M0partial_par"/1(q_m), M0mpartial_par/1(q_m)
  Lm_partial/1 -> Mmpartial/5(Lm_partial), M0mpartial/8(Lm_partial), M0mpartial_par/8(Lm_partial)

== matlab function temp_mmms4th/Controller4/Nullspace_maps ==
  data: Mm input; A input; N output; q_dot_m input
function N  =Nullspace_maps(Mm,A,q_dot_m)

n=length(q_dot_m);

N_Am=eye(n)-(Mm\A') *   (   (   (A/Mm) *   A')\    A);
N=N_Am;

== matlab function temp_mmms4th/Controller4/Potential Function ==
  data: U_ff output; A input; w input; grad_w input; U_c input; p_0n input; sc_size input; Mm_hat input; g_n0 input
function U_ff = U_ff(A,w,grad_w, U_c, p_0n, sc_size,Mm_hat, g_n0)


grad_w_p=p_0n/(norm(p_0n)); % d/dt(1/sqrt(x^2+y^2+z^2)) = -1/2*w_p^3 * d/dt (x^2+...)
w_lim=0.003;
w_p_lim=0.02;
r_lim=sqrt(2)*sc_size/2+0.02;

w_p=norm(p_0n)-r_lim;

JJ=A;
A_dagger = ((Mm_hat)\JJ')/((JJ/Mm_hat)*JJ');

if w<w_lim %--------------------------------------------- close to singular
%     temp=(pinv(A)'*grad_w);
%     dir=(temp)./(norm(temp));
%     Uc=U_c-dot(U_c,dir).*dir;

    if w_p<w_p_lim %-------------- EE collision w Spacecraft
        if w_p<w_p_lim/4
            U_c=U_c;
        end
        U_c=U_c;%-10.*(1-w_p_lim/w_p)*((w_p_lim)/w_p^2).*[(grad_w_p); zeros(3,1)]; %(1/(1+100*exp(1000*(w_p-(sqrt(2)*sc_size/2+0.05)))))*2*
    end
    
    U_ff=U_c-((1-w_lim/w)*(w_lim/w^2).*A_dagger'*grad_w); %1*(1-w_lim/w)*
    %(1/(1+100*exp(1000*(w-0.003))))*0.0001*pinv(A)'*(-grad_w./(w^2)); 
    %adjoint_low(Adjoint(g_I0)*V_Ie)*Adjoint(inv(g_I0))*V_It+Adjoint(inv(g_I0))*V_It_dot

else %----------------------------------------------- NOT close to singular
    
    if w_p<w_p_lim %-------------- EE collision w Spacecraft
        if w_p<w_p_lim/4
            U_c=U_c-dot(U_c,[(grad_w_p); zeros(3,1)]);
        end
        U_c=U_c;%-10.*(1-w_p_lim/w_p)*((w_p_lim)/w_p^2).*[(grad_w_p); zeros(3,1)];
        %(1/(1+100*exp(1000*(w_p-(sqrt(2)*sc_size/2+0.05)))))*2*
        
    end

    U_ff=U_c;
end

== matlab function temp_mmms4th/Controller4/Potential Function1 ==
  data: w_p output; p_0n input
function w_p = norm( p_0n)

w_p=norm(p_0n);

== matlab function temp_mmms4th/Controller4/Potential Function3 ==
  data: f_pot output; p_ni input; g_ni input; sc_size input; g_n0 input; A input; p_i output; unirand input
function [f_pot,p_i]  = potential_joints( p_ni, g_ni, sc_size, g_n0, A, unirand)

% w_joints=zeros(1,4);
grad_p_joints=zeros(3,4);
grad_p=zeros(7,4);
f_pot=zeros(7,1);
gain=0.01.*[1 1 1 1];%*[70 70 70 70];

p_lim=0.05;
r_lim=sqrt(2)*sc_size/2;


p_i=[0;0;0;0];

alpha_fraction=0.1;

for i=1:4
    noise = unirand.* (alpha_fraction .* p_i(i));
    p_i(i)=p_i(i)+noise;

    p_i(i)=norm(p_ni(:,i))-r_lim; %X_e
end

J_joints=zeros(4,7,6);
tempj=zeros(4,4);
for i=1:4
    % J_joints(i,:,:)=Adjoint(inv(g_n0))*[A(:,1:i+1) 0.*A(:,i+2:end)];
    tempj(:,:)=g_ni(i,:,:);
    J_joints(i,:,:)=[0.*A(:,1:i+1) -A(:,i+2:end)]'*Adjoint(inv(g_n0\tempj))';
end

R=zeros(3,3);
temp=zeros(7,6);
norm_grad_p=zeros(4,1);
% temp2=zeros(4);
    for i=1:4 %------------------------------ Joints collision w Spacecraft
        % w_joints(i)=norm(p_joints(:,i));%+[0; 0; 0.15]);
        if p_i(i)>p_lim %|| p_i<0.001
            grad_p_joints(:,i)=zeros(3,1);
        elseif p_i(i)<=0 && p_i(i)>-p_lim
            grad_p_joints(:,i)=-(p_ni(:,i))/norm(p_ni(i));
        elseif p_i(i)<-p_lim
            grad_p_joints(:,i)=zeros(3,1);
        else
            grad_p_joints(:,i)=(p_ni(:,i))/norm(p_ni(i));
        end
        temp(:,:)=J_joints(i,:,:);
        
        % temp2=squeeze(g_ni(i,:,:));
        % temp3=g_n0*temp2;

        R(:,:)=g_ni(i,1:3,1:3);
        grad_p(:,i)=temp*[R'*grad_p_joints(:,i);zeros(3,1)];
        norm_grad_p(i)=norm(grad_p(:,i));
        
    
        if p_i(i)<p_lim
            f_pot=f_pot-gain(i)*(1-p_lim/p_i(i))*((p_lim)/(p_i(i))^2).*(grad_p(:,i));  %((1/(1+100*exp(1000*(-(sqrt(2)*sc_size/2+0.0)))))
        end
        
    end

== matlab function temp_mmms4th/Controller4/V_It_1 ==
  data: V_It input; g_It input; V_It_3 output
function V_It_3 = V_It3(V_It, g_It)


% g_gpt=[eye(3) [0.25; 0.25; 0.25]; 0 0 0 1];
R=g_It(1:3,1:3);

V_It_3=Adjoint(g_It)*[R zeros(3);zeros(3) R]'*V_It; %[R zeros(3);zeros(3) R]


% Ad g_Igp(t) M^-1 Ad gI_gp(t)' inv(Ad g_I_gp') Mt inv (Ad g_I_gp) V_Igp

== matlab function temp_mmms4th/Controller4/V_It_2 ==
  data: mu_t input; M_t_body input; g_It input; V_It_2 output
function V_It_2 = V_It(mu_t, M_t_body, g_It)


% g_gpt=[eye(3) [0.25; 0.25; 0.25]; 0 0 0 1];
R=g_It(1:3,1:3);

% Pt=(Adjoint(g_It))'*mu_t;
V_It_2=(Adjoint(g_It))*inv(M_t_body)*(Adjoint(g_It)')*mu_t;%Adjoint(g_It)*M_t_body\Pt;%(Mt\(Adjoint(g_It)')*Pt); %[R zeros(3);zeros(3) R]



% Ad g_Igp(t) M^-1 Ad gI_gp(t)' inv(Ad g_I_gp') Mt inv (Ad g_I_gp) V_Igp

== matlab function temp_mmms4th/Controller4/Velocity_error1 ==
  data: w input; out output; in input
function out = cut_off(w, in)

if w<0.003
    out=0.*in; %adjoint_low(Adjoint(g_I0)*V_Ie)*Adjoint(inv(g_I0))*V_It+Adjoint(inv(g_I0))*V_It_dot
else
    out=in;
end

== matlab function temp_mmms4th/Controller4/Z ==
  data: N input; Z output; Z_dagger output; Mm input; j output; Nj output
function [Z,Z_dagger,j,Nj] =Z(N,Mm)

% m=length(temp(1,:));
% 
% for i=1:m
%     Z(:,i)=Mm*temp(:,i);
% end
nN=zeros(7,1);
for j=1:7
    nN(j,1)=N(:,j)'*N(:,j);
end

[nmax,j]=max(nN);

Z=N(:,j)/norm(N(:,j));

Z_dagger=(Z'*Mm*Z)\(Z'*Mm);

norm_Z=norm(N(:,j));

Nj=N(:,j);

== matlab function temp_mmms4th/Controller4/Z dagger derivative ==
  data: Z_dagger input; N_dot input; Z_dot_dagger output; Z_dot input
function Z_dot_dagger =Z_dot_dagger(Z_dagger,N_dot,Z_dot)

Z_dot_dagger=Z_dagger*N_dot-Z_dagger*Z_dot*Z_dagger;

== matlab function temp_mmms4th/Controller4/ZKw ==
  data: Z input; K_w_grad_w input; out output
function out  =for_i(Z, K_w_grad_w)


out=Z'*K_w_grad_w;

== matlab function temp_mmms4th/Controller4/grad w ==
  data: A input; grad_w output; A_partial input; q_dot input
function grad_w  = grad_w(A,A_partial, q_dot)

w=sqrt(det(A*A'));

n=length(q_dot);
grad_w=zeros(n,1);
for i=1:n
    grad_w(i) = w/2* trace(   (A*A')\(A*A_partial(:,:,i)'+A_partial(:,:,i)*A')    );%det(A*A')*trace(inv(A')A_dot'+inv(A')*inv(A)*A_dot*A');
end

% w_dot=1/norm(grad_w'*q_dot);

== matlab function temp_mmms4th/Controller4/gradient_of_Eg ==
  data: g_te input; Nabla_Eg output
function Nabla_Eg = fcn(g_te)

% Calculate the gradient of the Pose Error Function
p_te=g_te(1:3,4);
R_te=g_te(1:3,1:3);

temp=0.5*(R_te-transpose(R_te));

R_temp=vee3(temp);

Nabla_Eg=[p_te;R_temp];

== matlab function temp_mmms4th/Controller4/joint distance from spacecraft ==
  data: pnorm output; p_joints input
function pnorm = norm( p_joints)

pnorm=zeros(4,1);
for i=1:4
    pnorm(i)=norm(p_joints(:,i));
end

== matlab function temp_mmms4th/Controller4/mu_init ==
  data: g_It input; Mt input; V_It input; mu_init output
function mu_init = mu_init(g_It,Mt,V_It)

mu_init=Mt*V_It; %*(inv(Adjoint(g_It)))


% Ad g_Igp(t) M^-1 Ad gI_gp(t)' inv(Ad g_I_gp') Mt inv (Ad g_I_gp) V_Igp

== matlab function temp_mmms4th/Controller4/nullspace_mapping ==
  data: Mm input; K_w_grad_w input; q_dot_m input; Z input; Z_dagger input; f_N output; Z_dot_dagger input; K_nu_nu input; f_pot input; out2 output; fw_i input
function [f_N, out2] =null_space(Mm, K_w_grad_w, q_dot_m,Z, Z_dagger,Z_dot_dagger, K_nu_nu, f_pot, fw_i)

f_N=zeros(7,1);

% nu=Z_dagger*q_dot_m;


f_N=Mm*Z*(-Z_dot_dagger*q_dot_m-K_nu_nu+1.*Z'*K_w_grad_w-0.*fw_i +Z_dagger*f_pot);

out2=Z_dagger*K_w_grad_w;

% 
% for i=1:m
%     fw =fw+ dot(w_opt, null_space(:,i)) / norm(null_space(:,i))^2 * null_space(:,i);
% end

% for i=1:m
%     fw =fw+ dot(f_pot, null_space(:,i)) / norm(null_space(:,i))^2 * null_space(:,i);
% end

% A_dot=A_partial*q_dot;


% JJ=A/Mm;
% null_space=eye(7)-(JJ'/(JJ*JJ'))*JJ;
% fw=zeros(7,1);
% fw=fw+null_space*f_pot;
% f_N=fw+null_space*w_opt;

== matlab function temp_mmms4th/Feedback Transformation3/Inverse Dynamics1/A_dot ==
  data: A_partial input; q_m_dot input; A_dot output
function A_dot = fcn(A_partial, q_m_dot)
n=length(q_m_dot);

A_dot=zeros(6,n);
for i=1:n
    A_dot=A_dot+A_partial(:,:,i).*q_m_dot(i);
end

== matlab function temp_mmms4th/Feedback Transformation3/Inverse Dynamics1/C_hat/AMA_partial ==
  data: q_m input; AMA_partial output; M0 input; A input; A_partial input; V input; M0_partial input
function AMA_partial = AMA_partial(q_m,M0,A,A_partial,V,M0_partial)
% Calculates the C_hat_m matrix from base pose and arm joint angles

n=length(q_m);
b=length(V);

% find the temp intermediate term
AMA_partial=zeros(n,n,n);
for i=1:n
    AMA_partial(1:n,1:n,i)=transpose(A_partial(1:end,1:end,i))*M0*A+transpose(A)*M0_partial(1:end,1:end,i)*A+transpose(A)*M0*A_partial(1:end,1:end,i); %calcualte the derivative of not-augmented arm mass matrix from equation 121 of TRO paper
end

== matlab function temp_mmms4th/Feedback Transformation3/Inverse Dynamics1/C_hat/A_partial ==
  data: q_m input; A_partial output; M0 input; M0_partial input; M0m_partial input; M0m input; V input
function A_partial = A_partial(q_m,M0,M0_partial,M0m_partial,M0m,V)
% Calculates the C_hat_m matrix from base pose and arm joint angles

n=length(q_m);
b=length(V);

% Find partial of connection A to each joint angle
A_partial=zeros(b,n,n);

temp1=zeros(b,n);
temp2=zeros(b,n);
temp3=zeros(b,n);

for i=1:n
    temp1=M0\(M0_partial(:,:,i));
    temp2=M0\M0m;
    temp3=M0\(M0m_partial(:,:,i));
    A_partial(1:b,1:n,i)=-temp1*temp2+temp3; % Equation 122
end

== matlab function temp_mmms4th/Feedback Transformation3/Inverse Dynamics1/C_hat/C_hat1 ==
  data: q_m input; Mm_hat_partial input; q_dot_m input; C_hat output
function C_hat = C_hat(q_m, Mm_hat_partial,q_dot_m)
% Calculates the C_hat_m matrix from base pose and arm joint angles

n=length(q_m);


% Calculate C_hat matrix
C_temp1=zeros(n,n);
C_temp2=zeros(n,n);
C_hat=zeros(n,n);
for i=1:n
    C_temp1=C_temp1+squeeze(Mm_hat_partial(1:n,1:n,i)).*q_dot_m(i); % nxn by scalar
    C_temp2(i,1:n)=0.5*transpose(q_dot_m)*squeeze(Mm_hat_partial(1:n,1:n,i)); %1xn by nxn 
end

C_hat=C_temp1-C_temp2;

== matlab function temp_mmms4th/Feedback Transformation3/Inverse Dynamics1/C_hat/Lm_partials/Lm0partial ==
  data: q_m input; Lm0_partial output; Xi_m input; iota0 input
function Lm0_partial = Lm0_partial(q_m,Xi_m,iota0)
% Calculates the C_hat_m matrix from base pose and arm joint angles

n=length(q_m);

% Find partial of Lm to joint angles
Lm0_partial=zeros(6*n,6,n); % 6nx6xn
for i=1:n
    for j=1:n
        Lm0_partial(6*(j-1)+1:6*j,1:6,i)=Ad_partial(j,1,i,Xi_m,q_m,iota0); % equation 114 of TRO paper
    end
end

%%%%%%%%%%%%%%%%%%%%%%%%%%%%%%%%%%%%%%%%%%%%%%%%%%%%%%%%%%%%% MUST BE
%%%%%%%%%%%%%%%%%%%%%%%%%%%%%%%%%%%%%%%%%%%%%%%%%%%%%%%%%%%%% CHECKED

== matlab function temp_mmms4th/Feedback Transformation3/Inverse Dynamics1/C_hat/Lm_partials/Lmpartial ==
  data: q_m input; Lm_partial output; Xi_m input; iota0 input
function Lm_partial  = Lm_partial(q_m,Xi_m,iota0)
% Calculates the C_hat_m matrix from base pose and arm joint angles

n=length(q_m);

% Find partial of Lm0 to joint angles
Lm_partial=zeros(6*n,6*n,n); % 6nx6xn
for i=1:n
    Lm_partial(:,:,i)=zeros(6*n,6*n);
    for j=2:n
        for k=2:n
            if j>i && i>=k
                Lm_partial(6*(j-1)+1:6*j,6*(k-2)+1:6*(k-1),i)=Ad_partial(j,k,i,Xi_m,q_m,iota0); % equation 81 of TRO paper
            elseif i==j && i>=k
                Lm_partial(6*(j-1)+1:6*j,6*(k-2)+1:6*(k-1),i)=Ad_partial(j,k,i,Xi_m,q_m,iota0); % equation 81 of TRO paper
            else
                Lm_partial(6*(j-1)+1:6*(j-1)+6,6*(k-2)+1:6*(k-2)+6,i)=zeros(6,6);
            end

        end
    end
end

== matlab function temp_mmms4th/Feedback Transformation3/Inverse Dynamics1/C_hat/M_partials/ M0partial ==
  data: q_m input; M0_partial output; Lm0 input; V input; iota0 input; diag_Mm input; Lm0_partial input
function M0_partial = M0_partial(q_m,Lm0,V,iota0,diag_Mm,Lm0_partial)
% Calculates the C_hat_m matrix from base pose and arm joint angles

n=length(q_m);
b=length(V);

% Find partial of M0 to joint angles
M0_partial=zeros(b,b,n); %initiate
for i=1:n
    temp1=transpose(Lm0_partial(1:end,1:end,i))*diag_Mm*Lm0;
    temp2=transpose(Lm0)*diag_Mm*Lm0_partial(1:end,1:end,i);
    M0_partial(1:b,1:b,i)= iota0'*(temp1+temp2)*iota0; %6x6 %equation 117 of TRO
end

== matlab function temp_mmms4th/Controller4/  ==
  data: A input; normA output
function normA  = normA(A)

normA=norm(A);

== matlab function temp_mmms4th/Feedback Transformation3/Inverse Dynamics1/C_hat/M_partials/M0mpartial ==
  data: q_m input; M0m_partial output; V input; Lm input; Lm0 input; iota0 input; diag_Mm input; Lm0_partial input; Lm_partial input; Xi_m_matrix input
function M0m_partial = M0m_partial(q_m,V,Lm,Lm0,iota0,diag_Mm,Lm0_partial,Lm_partial, Xi_m_matrix)
% Calculates the C_hat_m matrix from base pose and arm joint angles

n=length(q_m);
b=length(V);

% Find partial of M0m to joint angles
M0m_partial=zeros(b,n,n);
for i=1:n
    temp1=transpose(Lm0_partial(1:end,1:end,i))*diag_Mm*Lm;
    temp2=transpose(Lm0)*diag_Mm*Lm_partial(1:end,1:end,i);
    M0m_partial(1:b,1:n,i)= iota0'*(temp1+temp2)*Xi_m_matrix; % equation 118 of TRO paper
end

== matlab function temp_mmms4th/Feedback Transformation3/Inverse Dynamics1/C_hat/M_partials/Mmpartial ==
  data: q_m input; Mm_partial output; Xi_m_matrix input; Lm input; diag_Mm input; Lm_partial input
function Mm_partial = Mm_partial(q_m,Xi_m_matrix,Lm,diag_Mm,Lm_partial)
% Calculates the C_hat_m matrix from base pose and arm joint angles

n=length(q_m);

% find the non-generalized arm mass matrix'x derivative to joint angles
Mm_partial=zeros(n,n,n);
for i=1:n
    temp=   transpose(Lm_partial(1:6*n,1:6*n,i))*diag_Mm*Lm  +   transpose(Lm)*diag_Mm*Lm_partial(1:6*n,1:6*n,i);
    Mm_partial(1:n,1:n,i)=transpose(Xi_m_matrix)*temp*Xi_m_matrix; %calcualte the derivative of not-augmented arm mass matrix from equation 120 of TRO paper
end

== matlab function temp_mmms4th/Feedback Transformation3/Inverse Dynamics1/C_hat/Mm_hat_partial ==
  data: q_m input; AMA_partial input; Mm_hat_partial output; Mm_partial input
function Mm_hat_partial = Mm_hat_partial(q_m, AMA_partial, Mm_partial)
% Calculates the C_hat_m matrix from base pose and arm joint angles

n=length(q_m);

% find the generalized arm mass matrix'x derivative to joint angles
Mm_hat_partial=zeros(n,n,n);
for i=1:n
    Mm_hat_partial(1:n,1:n,i)=Mm_partial(1:n,1:n,i)-AMA_partial(1:n,1:n,i); %calcualte the derivative of augmented arm mass matrix from equation 119 of TRO paper
end

== matlab function temp_mmms4th/Feedback Transformation3/Inverse Dynamics1/C_hat1/AMA_partial1 ==
  data: q_m input; AMA_partial output; M0 input; A input; A_partial input; V input; M0_partial input
function AMA_partial = AMA_partial(q_m,M0,A,A_partial,V,M0_partial)
% Calculates the C_hat_m matrix from base pose and arm joint angles

n=length(q_m);
b=length(V);

% find the temp intermediate term
AMA_partial=zeros(n,n,n);
for i=1:n
    AMA_partial(1:n,1:n,i)=transpose(A_partial(1:end,1:end,i))*M0*A+transpose(A)*M0_partial(1:end,1:end,i)*A+transpose(A)*M0*A_partial(1:end,1:end,i); %calcualte the derivative of not-augmented arm mass matrix from equation 121 of TRO paper
end

== matlab function temp_mmms4th/Feedback Transformation3/Inverse Dynamics1/C_hat1/A_partial1 ==
  data: q_m input; A_partial output; M0 input; M0_partial input; M0m_partial input; M0m input; V input
function A_partial = A_partial(q_m,M0,M0_partial,M0m_partial,M0m,V)
% Calculates the C_hat_m matrix from base pose and arm joint angles

n=length(q_m);
b=length(V);

% Find partial of connection A to each joint angle
A_partial=zeros(b,n,n);

temp1=zeros(b,n);
temp2=zeros(b,n);
temp3=zeros(b,n);

for i=1:n
    temp1=M0\M0_partial(1:end,1:end,i);
    temp2=M0\M0m;
    temp3=M0\M0m_partial(1:end,1:end,i);
    A_partial(1:b,1:n,i)=-temp1*temp2+temp3; % Equation 122
end

== matlab function temp_mmms4th/Feedback Transformation3/Inverse Dynamics1/C_hat1/A_partial_par ==
  data: q_m input; A_partial_par output; M0 input; M0_partial input; M0m_partial input; M0m input; V input; M0_partial_par input; M0m_partial_par input
function A_partial_par = A_partial_par(q_m,M0,M0_partial,M0m_partial,M0m,V,M0_partial_par,M0m_partial_par)
% Calculates the C_hat_m matrix from base pose and arm joint angles

n=length(q_m);
b=length(V);

% Find partial of connection A to each joint angle
A_partial_par=zeros(b,n,n,n);

temp1=zeros(b,n);
temp2=zeros(b,n);
temp3=zeros(b,n);

for i=1:n
    for s=1:n
        temp1=M0\M0_partial(1:end,1:end,i);
        temp2=M0\M0_partial(1:end,1:end,s);
        temp3=M0\M0m;
        temp4=M0\M0m_partial(1:end,1:end,i);
        temp5=M0\M0m_partial(1:end,1:end,s);
        A_partial_par(1:b,1:n,i,s)=(M0\     (M0_partial(1:end,1:end,s)*temp1 -M0_partial_par(1:end,1:end,i,s) +M0_partial(1:end,1:end,i)*temp2)           )*temp3 ...
            +M0\(-M0_partial(1:end,1:end,i)*temp5-M0_partial(1:end,1:end,s)*temp4+M0m_partial_par(1:end,1:end,i,s)); % Equation 122????????
    end 
end

== matlab function temp_mmms4th/Controller4/CBF ==
  data: w input; grad_w input; CBF output; Mm_hat input; f_m input; C_hat input; N_hat input; Hes_w input; q_dot input; h_ddot output
function [CBF,h_ddot] = CBF(w,grad_w,Mm_hat,f_m,C_hat,N_hat,Hes_w,q_dot)

n=length(q_dot);


h_ddot=grad_w'*(Mm_hat\(f_m-C_hat*q_dot-N_hat))+q_dot'*Hes_w'*q_dot;

psi=grad_w'*(Mm_hat\(f_m-C_hat*q_dot-N_hat))+q_dot'*Hes_w*q_dot+20*grad_w'*q_dot+100*(w-0.003);

if psi<0
    CBF=-Mm_hat*grad_w.*(psi/(grad_w'*grad_w)); %adjoint_low(Adjoint(g_I0)*V_Ie)*Adjoint(inv(g_I0))*V_It+Adjoint(inv(g_I0))*V_It_dot
else
    CBF=zeros(n,1);
end

== matlab function temp_mmms4th/Feedback Transformation3/Inverse Dynamics1/C_hat1/C_hat2 ==
  data: q_m input; Mm_hat_partial input; q_dot_m input; C_hat output
function C_hat = C_hat(q_m, Mm_hat_partial,q_dot_m)
% Calculates the C_hat_m matrix from base pose and arm joint angles

n=length(q_m);


% Calculate C_hat matrix
C_temp1=zeros(n,n);
C_temp2=zeros(n,n);
C_hat=zeros(n,n);
for i=1:n
    C_temp1=C_temp1+squeeze(Mm_hat_partial(1:n,1:n,i)).*q_dot_m(i); % nxn by scalar
    C_temp2(i,1:n)=0.5*transpose(q_dot_m)*squeeze(Mm_hat_partial(1:n,1:n,i)); %1xn by nxn 
end

C_hat=C_temp1-C_temp2;

== matlab function temp_mmms4th/Feedback Transformation3/Inverse Dynamics1/C_hat1/Lm_partials1/Lm0partial ==
  data: q_m input; Lm0_partial output; Xi_m input; iota0 input
function Lm0_partial = Lm0_partial(q_m,Xi_m,iota0)
% Calculates the C_hat_m matrix from base pose and arm joint angles

n=length(q_m);

% Find partial of Lm to joint angles
Lm0_partial=zeros(6*n,6,n); % 6nx6xn
for i=1:n
    for j=1:n
        Lm0_partial(6*(j-1)+1:6*j,1:6,i)=Ad_partial(j,1,i,Xi_m,q_m,iota0); % equation 114 of TRO paper
    end
end

%%%%%%%%%%%%%%%%%%%%%%%%%%%%%%%%%%%%%%%%%%%%%%%%%%%%%%%%%%%%% MUST BE
%%%%%%%%%%%%%%%%%%%%%%%%%%%%%%%%%%%%%%%%%%%%%%%%%%%%%%%%%%%%% CHECKED
